simulink library "deadtime_with_minimum_pulse_generator"  (R2025b)
settings: Solver=VariableStepAuto  StartTime=0.0  StopTime=10.0  RelTol=1e-3
libraries: ee_lib x114, fl_lib x20, nesl_utility x5
(part 1 of 12)
settings Model: Creator=dbagn  LastModifiedBy=dbagn

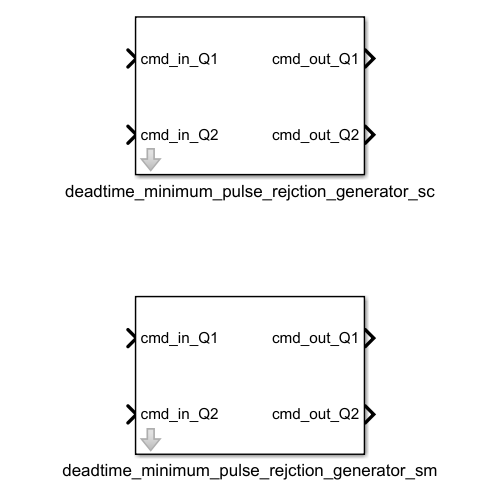
[thumbnail: Simulink's stored preview of the top-level diagram]
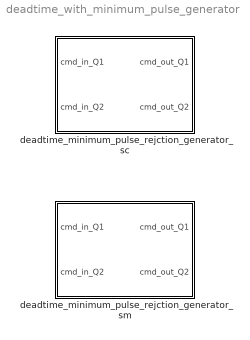
== system deadtime_with_minimum_pulse_generator ==
  deadtime_minimum_pulse_rejction_generator_sc : Subsystem  mask{Vpos_rail_dtg=15, Vneg_rail_dtg=0, Cdt=820e-12, Rdt=3.3e3, Cmp=270e-12, Rmp=3.3e3}
      mask prompts: Vpos_rail_dtg "Positive Voltage Rail Supply"; Vneg_rail_dtg "Negative Voltage Rail Supply"; Cdt "C dead time [F]"; Rdt "R dead time [Ohm]"; Cmp "C min pulse [F]"; Rmp "R min pulse [Ohm]"
  deadtime_minimum_pulse_rejction_generator_sm : Subsystem  mask{Vpos_rail_dtg=12, deadtime=2e-6, minimum_pulse=2e-6}
      mask prompts: Vpos_rail_dtg "Positive Voltage Rail Supply"; deadtime "DeadTime [s]"; minimum_pulse "Minimum Pulse [s]"

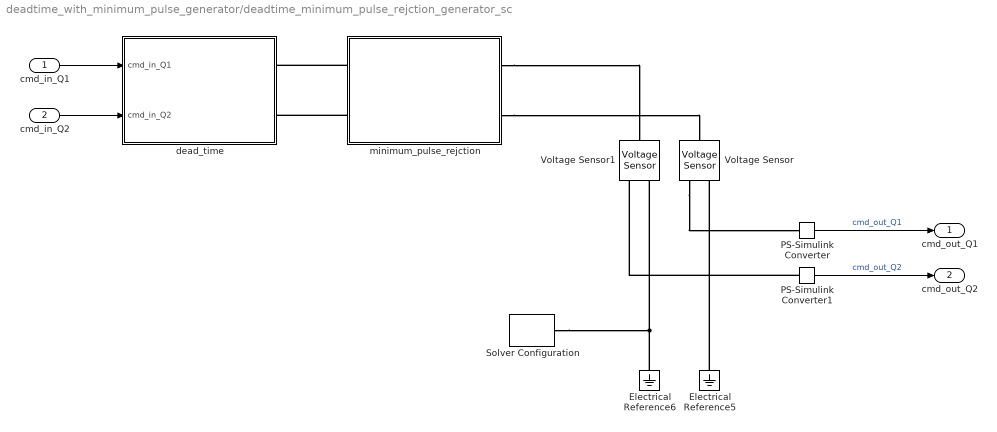
== system deadtime_with_minimum_pulse_generator/deadtime_minimum_pulse_rejction_generator_sc ==
  cmd_in_Q1 : Inport
  cmd_in_Q2 : Inport  Port=2
  Electrical Reference5 : fl_lib/Electrical/Electrical Elements/Electrical Reference
  Electrical Reference6 : fl_lib/Electrical/Electrical Elements/Electrical Reference
  PS-Simulink Converter : nesl_utility/PS-Simulink Converter  PhysicalDomain=network_engine_domain  SubClassName=ps_output  LeftPortType=input  RightPortType=output  PseudoPeriodic=off  Frequencies=[]  VectorFormat=1-D array  Unit=V  AffineConversion=off
  PS-Simulink Converter1 : nesl_utility/PS-Simulink Converter  PhysicalDomain=network_engine_domain  SubClassName=ps_output  LeftPortType=input  RightPortType=output  PseudoPeriodic=off  Frequencies=[]  VectorFormat=1-D array  Unit=V  AffineConversion=off
  Solver Configuration : nesl_utility/Solver Configuration  PhysicalDomain=network_engine_domain  SubClassName=solver  LeftPortType=input  RightPortType=generic  Tones=[]  Harmonics=[]  SimulateNoise=off  Profile=off  UseLocalSampling=off  EnableSwitchedLinearOptims=on  FrequencyDomain=off  UseCCode=off  RelTol=0.001  AbsTol=0.001  MinStep=1e-09  ToWorkspace=off  RevertToSquareIcSolve=off  NumHomotopyIterations=100  PhasorMode=off  PhasorModeNumHarmonics=1  ConsistencySolver=NEWTON_XTOL_AFTER_FTOL  IndexReductionMethod=DerivativeReplacement  DoDC=on  ResidualTolerance=1e-09  ConsistencyTolSource=GLOBAL  ConsistencyAbsTol=0.001  ConsistencyRelTol=0.001  ConsistencyTolFactor=0.001  UseLocalSolver=on  LocalSolverChoice=NE_BACKWARD_EULER_ADVANCER  ResolveIndetEquations=on  FunctionEvalNumThread=1  LocalSolverSampleTime=tc  DoFixedCost=off  MaxNonlinIter=5  MaxModeIter=2  ComputeImpulses=off  ImpulseIterations=2  LinearAlgebra=auto  LinearAlgebraNumThread=0  EquationFormulation=NE_TIME_EF  DelaysMemoryBudget=1024  AutomaticFiltering=on  FilteringTimeConstant=0.001  PartitionStorageMethod=AS_NEEDED  PartitionMemoryBudget=1024  PartitionMethod=ROBUST  MultibodyUseLocalSolver=off  MultibodyLocalSolverChoice=ODE1  MultibodyLocalSolverSampleTime=0.001
  Voltage Sensor : fl_lib/Electrical/Electrical Sensors/Voltage Sensor
  Voltage Sensor1 : fl_lib/Electrical/Electrical Sensors/Voltage Sensor
  dead_time : Subsystem
  minimum_pulse_rejction : Subsystem
  cmd_out_Q1 : Outport
  cmd_out_Q2 : Outport  Port=2
  wires:
  cmd_in_Q1/1 -> dead_time/1(cmd_in_Q1)
  cmd_in_Q2/1 -> dead_time/2(cmd_in_Q2)
  PS-Simulink Converter/1 -> cmd_out_Q1/1  "cmd_out_Q1"
  PS-Simulink Converter1/1 -> cmd_out_Q2/1  "cmd_out_Q2"
  connections:
  Electrical Reference6/LConn1 -- Voltage Sensor1/RConn2 -- Solver Configuration/RConn1
  Electrical Reference5/LConn1 -- Voltage Sensor/RConn2
  Voltage Sensor/RConn1 -- PS-Simulink Converter/LConn1
  PS-Simulink Converter1/LConn1 -- Voltage Sensor1/RConn1
  minimum_pulse_rejction/RConn1 -- Voltage Sensor1/LConn1
  minimum_pulse_rejction/RConn2 -- Voltage Sensor/LConn1
  minimum_pulse_rejction/LConn1 -- dead_time/RConn1
  minimum_pulse_rejction/LConn2 -- dead_time/RConn2

== system deadtime_with_minimum_pulse_generator/deadtime_minimum_pulse_rejction_generator_sm ==
  cmd_in_Q1 : Inport
  cmd_in_Q2 : Inport  Port=2
  dead_time : Subsystem
  minimum_pulse : Subsystem
  cmd_out_Q1 : Outport
  cmd_out_Q2 : Outport  Port=2
  wires:
  cmd_in_Q1/1 -> dead_time/1(cmd_in_Q1)
  cmd_in_Q2/1 -> dead_time/2(cmd_in_Q2)
  dead_time/1(cmd_out_Q1) -> minimum_pulse/1(cmd_in_Q1)
  dead_time/2(cmd_out_Q2) -> minimum_pulse/2(cmd_in_Q2)
  minimum_pulse/1(cmd_out_Q1) -> cmd_out_Q1/1
  minimum_pulse/2(cmd_out_Q2) -> cmd_out_Q2/1

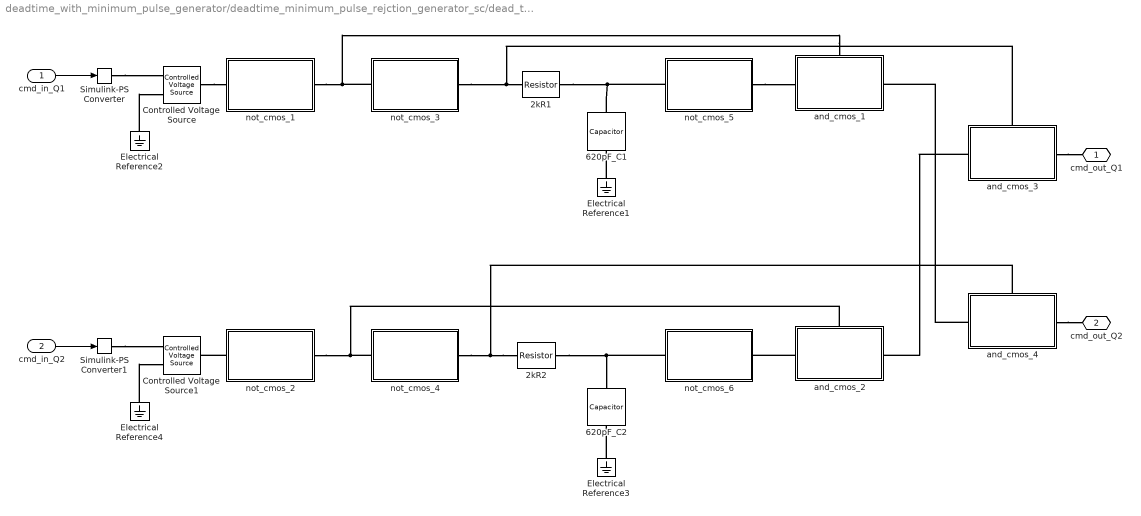
== system deadtime_with_minimum_pulse_generator/deadtime_minimum_pulse_rejction_generator_sc/dead_time ==
  cmd_in_Q1 : Inport
  cmd_in_Q2 : Inport  Port=2
  2kR1 : fl_lib/Electrical/Electrical Elements/Resistor  R=Rdt Ohm  i_specify=off  i_priority=None  i=0 A  i_nominal_specify=off  i_nominal_value=1  i_nominal_unit=A  v_specify=off  v_priority=None  v=0 V  v_nominal_specify=off  v_nominal_value=1  v_nominal_unit=V
  2kR2 : fl_lib/Electrical/Electrical Elements/Resistor  R=Rdt Ohm  i_specify=off  i_priority=None  i=0 A  i_nominal_specify=off  i_nominal_value=1  i_nominal_unit=A  v_specify=off  v_priority=None  v=0 V  v_nominal_specify=off  v_nominal_value=1  v_nominal_unit=V
  620pF_C1 : fl_lib/Electrical/Electrical Elements/Capacitor  c=Cdt F  r=1e-6 Ohm  g=0 1/Ohm  i_specify=off  i_priority=None  i=0 A  i_nominal_specify=off  i_nominal_value=1  i_nominal_unit=A  v_specify=off  v_priority=None  v=0 V  v_nominal_specify=off  v_nominal_value=1  v_nominal_unit=V  vc_specify=off  vc_priority=High  vc=0 V  vc_nominal_specify=off  vc_nominal_value=1  vc_nominal_unit=V
  620pF_C2 : fl_lib/Electrical/Electrical Elements/Capacitor  c=Cdt F  r=1e-6 Ohm  g=0 1/Ohm  i_specify=off  i_priority=None  i=0 A  i_nominal_specify=off  i_nominal_value=1  i_nominal_unit=A  v_specify=off  v_priority=None  v=0 V  v_nominal_specify=off  v_nominal_value=1  v_nominal_unit=V  vc_specify=off  vc_priority=High  vc=0 V  vc_nominal_specify=off  vc_nominal_value=1  vc_nominal_unit=V
  Controlled Voltage Source : fl_lib/Electrical/Electrical Sources/Controlled Voltage Source
  Controlled Voltage Source1 : fl_lib/Electrical/Electrical Sources/Controlled Voltage Source
  Electrical Reference{1..4} (4 alike) : fl_lib/Electrical/Electrical Elements/Electrical Reference
  Simulink-PS Converter : nesl_utility/Simulink-PS Converter  PhysicalDomain=network_engine_domain  SubClassName=ps_input  LeftPortType=input  RightPortType=output  PseudoPeriodic=off  Frequencies=[]  NoiseDistribution=none  NoiseParameters=[]  Unit=V  AffineConversion=off  FilteringAndDerivatives=provide  SimscapeFilterOrder=1  InputFilterTimeConstant=0.001  UdotUserProvided=0
  Simulink-PS Converter1 : nesl_utility/Simulink-PS Converter  PhysicalDomain=network_engine_domain  SubClassName=ps_input  LeftPortType=input  RightPortType=output  PseudoPeriodic=off  Frequencies=[]  NoiseDistribution=none  NoiseParameters=[]  Unit=V  AffineConversion=off  FilteringAndDerivatives=provide  SimscapeFilterOrder=1  InputFilterTimeConstant=0.001  UdotUserProvided=0
  and_cmos_1 : Subsystem
      settings: PortSchema="{\"entries\":[{\"content\":{\"sides\":[{\"content\":{\"connectorIds\":[\"LConn1\"]},\"type\":\"ConnectorPlacement.EquallySpacedRectSide\",\"uuid\":\"4468949f-f30a-49ce-949f-963bd607b697\"},{\"content\":{\"connectorIds\":[\"RConn1\"],\"side\":\"RIGHT\"},\"type\":\"ConnectorPlacement.EquallySpacedRectSide\",\"uuid\":\"ceda4040-901d-4fda-af9a-fc2c310617d8\"},{\"content\":{\"connectorIds\":[\"LConn2\"],\"side\":\"TOP\"},\"type\":\"ConnectorPlacement.EquallySpacedRectSide\",\"uuid\":\"3bda88a2-72eb-4af6-8d76-f1ae25008c8e\"}]},\"type\":\"ConnectorPlacement.EquallySpacedConnector\",\"uuid\":\"29371ddd-6b02-4938-80a9-3e3398458dce\"}],\"packageUris\":[\"http://schema.mathworks.com/mf0/Connector/R2020b\"],\"version\":\"1.0\"}"
  and_cmos_2 : Subsystem
      settings: PortSchema="{\"entries\":[{\"content\":{\"sides\":[{\"content\":{\"connectorIds\":[\"LConn1\"]},\"type\":\"ConnectorPlacement.EquallySpacedRectSide\",\"uuid\":\"4468949f-f30a-49ce-949f-963bd607b697\"},{\"content\":{\"connectorIds\":[\"RConn1\"],\"side\":\"RIGHT\"},\"type\":\"ConnectorPlacement.EquallySpacedRectSide\",\"uuid\":\"ceda4040-901d-4fda-af9a-fc2c310617d8\"},{\"content\":{\"connectorIds\":[\"LConn2\"],\"side\":\"TOP\"},\"type\":\"ConnectorPlacement.EquallySpacedRectSide\",\"uuid\":\"3bda88a2-72eb-4af6-8d76-f1ae25008c8e\"}]},\"type\":\"ConnectorPlacement.EquallySpacedConnector\",\"uuid\":\"29371ddd-6b02-4938-80a9-3e3398458dce\"}],\"packageUris\":[\"http://schema.mathworks.com/mf0/Connector/R2020b\"],\"version\":\"1.0\"}"
  and_cmos_3 : Subsystem
      settings: PortSchema="{\"entries\":[{\"content\":{\"sides\":[{\"content\":{\"connectorIds\":[\"LConn1\"]},\"type\":\"ConnectorPlacement.EquallySpacedRectSide\",\"uuid\":\"4468949f-f30a-49ce-949f-963bd607b697\"},{\"content\":{\"connectorIds\":[\"RConn1\"],\"side\":\"RIGHT\"},\"type\":\"ConnectorPlacement.EquallySpacedRectSide\",\"uuid\":\"ceda4040-901d-4fda-af9a-fc2c310617d8\"},{\"content\":{\"connectorIds\":[\"LConn2\"],\"side\":\"TOP\"},\"type\":\"ConnectorPlacement.EquallySpacedRectSide\",\"uuid\":\"3bda88a2-72eb-4af6-8d76-f1ae25008c8e\"}]},\"type\":\"ConnectorPlacement.EquallySpacedConnector\",\"uuid\":\"29371ddd-6b02-4938-80a9-3e3398458dce\"}],\"packageUris\":[\"http://schema.mathworks.com/mf0/Connector/R2020b\"],\"version\":\"1.0\"}"
  and_cmos_4 : Subsystem
      settings: PortSchema="{\"entries\":[{\"content\":{\"sides\":[{\"content\":{\"connectorIds\":[\"LConn1\"]},\"type\":\"ConnectorPlacement.EquallySpacedRectSide\",\"uuid\":\"4468949f-f30a-49ce-949f-963bd607b697\"},{\"content\":{\"connectorIds\":[\"RConn1\"],\"side\":\"RIGHT\"},\"type\":\"ConnectorPlacement.EquallySpacedRectSide\",\"uuid\":\"ceda4040-901d-4fda-af9a-fc2c310617d8\"},{\"content\":{\"connectorIds\":[\"LConn2\"],\"side\":\"TOP\"},\"type\":\"ConnectorPlacement.EquallySpacedRectSide\",\"uuid\":\"3bda88a2-72eb-4af6-8d76-f1ae25008c8e\"}]},\"type\":\"ConnectorPlacement.EquallySpacedConnector\",\"uuid\":\"29371ddd-6b02-4938-80a9-3e3398458dce\"}],\"packageUris\":[\"http://schema.mathworks.com/mf0/Connector/R2020b\"],\"version\":\"1.0\"}"
  not_cmos_1 : Subsystem
  not_cmos_2 : Subsystem
  not_cmos_3 : Subsystem
  not_cmos_4 : Subsystem
  not_cmos_5 : Subsystem
  not_cmos_6 : Subsystem
  cmd_out_Q1 : PMIOPort  Side=Right
  cmd_out_Q2 : PMIOPort  Port=2  Side=Right
  wires:
  cmd_in_Q2/1 -> Simulink-PS Converter1/1
  cmd_in_Q1/1 -> Simulink-PS Converter/1
  connections:
  2kR2/LConn1 -- and_cmos_4/LConn2 -- not_cmos_4/RConn1
  Electrical Reference1/LConn1 -- 620pF_C1/RConn1
  and_cmos_1/LConn2 -- not_cmos_3/LConn1 -- not_cmos_1/RConn1
  and_cmos_4/RConn1 -- cmd_out_Q2/RConn1
  2kR1/RConn1 -- not_cmos_5/LConn1 -- 620pF_C1/LConn1
  and_cmos_4/LConn1 -- and_cmos_1/RConn1
  and_cmos_2/LConn1 -- not_cmos_6/RConn1
  not_cmos_2/RConn1 -- and_cmos_2/LConn2 -- not_cmos_4/LConn1
  Electrical Reference4/LConn1 -- Controlled Voltage Source1/RConn2
  Electrical Reference3/LConn1 -- 620pF_C2/RConn1
  Simulink-PS Converter1/RConn1 -- Controlled Voltage Source1/RConn1
  2kR1/LConn1 -- and_cmos_3/LConn2 -- not_cmos_3/RConn1
  2kR2/RConn1 -- not_cmos_6/LConn1 -- 620pF_C2/LConn1
  not_cmos_5/RConn1 -- and_cmos_1/LConn1
  and_cmos_3/RConn1 -- cmd_out_Q1/RConn1
  not_cmos_2/LConn1 -- Controlled Voltage Source1/LConn1
  Electrical Reference2/LConn1 -- Controlled Voltage Source/RConn2
  Controlled Voltage Source/LConn1 -- not_cmos_1/LConn1
  and_cmos_3/LConn1 -- and_cmos_2/RConn1
  Simulink-PS Converter/RConn1 -- Controlled Voltage Source/RConn1

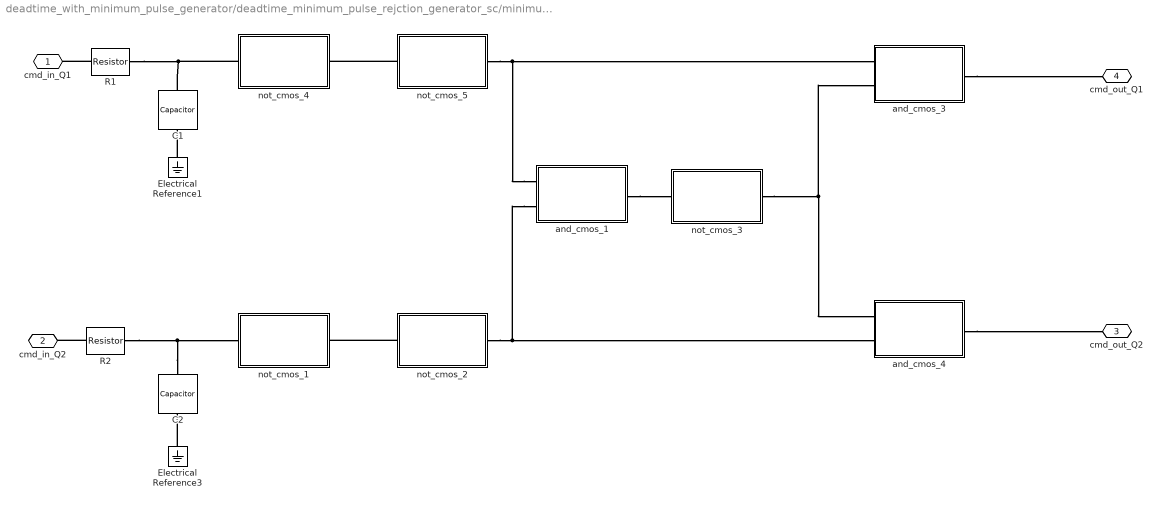
== system deadtime_with_minimum_pulse_generator/deadtime_minimum_pulse_rejction_generator_sc/minimum_pulse_rejction ==
  C1 : fl_lib/Electrical/Electrical Elements/Capacitor  c=Cmp F  r=1e-6 Ohm  g=0 1/Ohm  i_specify=off  i_priority=None  i=0 A  i_nominal_specify=off  i_nominal_value=1  i_nominal_unit=A  v_specify=off  v_priority=None  v=0 V  v_nominal_specify=off  v_nominal_value=1  v_nominal_unit=V  vc_specify=off  vc_priority=High  vc=0 V  vc_nominal_specify=off  vc_nominal_value=1  vc_nominal_unit=V
  C2 : fl_lib/Electrical/Electrical Elements/Capacitor  c=Cmp F  r=1e-6 Ohm  g=0 1/Ohm  i_specify=off  i_priority=None  i=0 A  i_nominal_specify=off  i_nominal_value=1  i_nominal_unit=A  v_specify=off  v_priority=None  v=0 V  v_nominal_specify=off  v_nominal_value=1  v_nominal_unit=V  vc_specify=off  vc_priority=High  vc=0 V  vc_nominal_specify=off  vc_nominal_value=1  vc_nominal_unit=V
  Electrical Reference1 : fl_lib/Electrical/Electrical Elements/Electrical Reference
  Electrical Reference3 : fl_lib/Electrical/Electrical Elements/Electrical Reference
  R1 : fl_lib/Electrical/Electrical Elements/Resistor  R=Rmp Ohm  i_specify=off  i_priority=None  i=0 A  i_nominal_specify=off  i_nominal_value=1  i_nominal_unit=A  v_specify=off  v_priority=None  v=0 V  v_nominal_specify=off  v_nominal_value=1  v_nominal_unit=V
  R2 : fl_lib/Electrical/Electrical Elements/Resistor  R=Rmp Ohm  i_specify=off  i_priority=None  i=0 A  i_nominal_specify=off  i_nominal_value=1  i_nominal_unit=A  v_specify=off  v_priority=None  v=0 V  v_nominal_specify=off  v_nominal_value=1  v_nominal_unit=V
  and_cmos_1 : Subsystem
  and_cmos_3 : Subsystem
  and_cmos_4 : Subsystem
  not_cmos_1 : Subsystem
  not_cmos_2 : Subsystem
  not_cmos_3 : Subsystem
  not_cmos_4 : Subsystem
  not_cmos_5 : Subsystem
  cmd_in_Q1 : PMIOPort  Side=Left
  cmd_in_Q2 : PMIOPort  Port=2  Side=Left
  cmd_out_Q2 : PMIOPort  Port=3  Side=Right
  cmd_out_Q1 : PMIOPort  Port=4  Side=Right
  connections:
  and_cmos_1/LConn1 -- and_cmos_3/LConn1 -- not_cmos_5/RConn1
  not_cmos_5/LConn1 -- not_cmos_4/RConn1
  and_cmos_1/RConn1 -- not_cmos_3/LConn1
  and_cmos_1/LConn2 -- and_cmos_4/LConn2 -- not_cmos_2/RConn1
  C2/LConn1 -- not_cmos_1/LConn1 -- R2/RConn1
  R1/RConn1 -- C1/LConn1 -- not_cmos_4/LConn1
  R1/LConn1 -- cmd_in_Q1/RConn1
  not_cmos_3/RConn1 -- and_cmos_4/LConn1 -- and_cmos_3/LConn2
  not_cmos_2/LConn1 -- not_cmos_1/RConn1
  Electrical Reference1/LConn1 -- C1/RConn1
  Electrical Reference3/LConn1 -- C2/RConn1
  and_cmos_3/RConn1 -- cmd_out_Q1/RConn1
  and_cmos_4/RConn1 -- cmd_out_Q2/RConn1
  R2/LConn1 -- cmd_in_Q2/RConn1

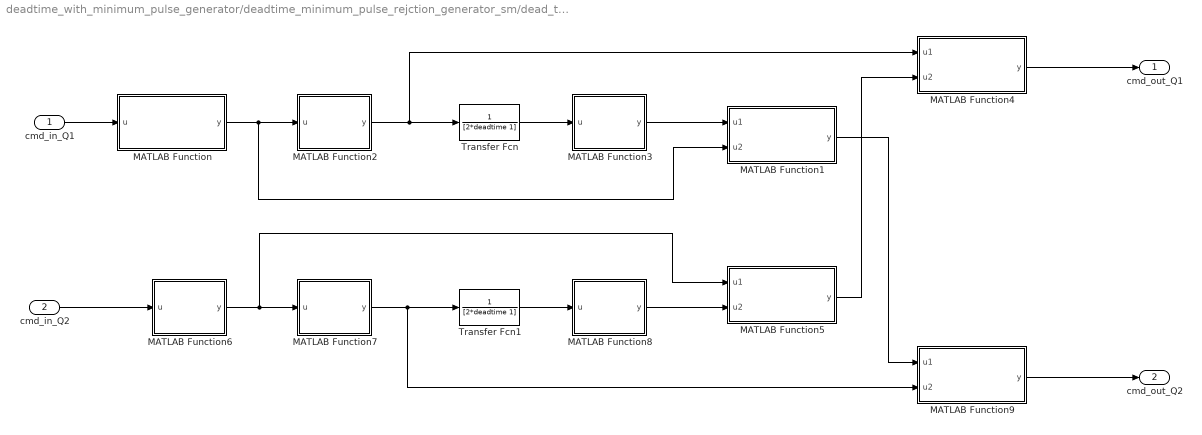
== system deadtime_with_minimum_pulse_generator/deadtime_minimum_pulse_rejction_generator_sm/dead_time ==
  cmd_in_Q1 : Inport
  cmd_in_Q2 : Inport  Port=2
  MATLAB Function : MATLAB Function  TreatAsAtomicUnit=on
  MATLAB Function1 : MATLAB Function  TreatAsAtomicUnit=on
  MATLAB Function2 : MATLAB Function  TreatAsAtomicUnit=on
  MATLAB Function3 : MATLAB Function  TreatAsAtomicUnit=on
  MATLAB Function4 : MATLAB Function  TreatAsAtomicUnit=on
  MATLAB Function5 : MATLAB Function  TreatAsAtomicUnit=on
  MATLAB Function6 : MATLAB Function  TreatAsAtomicUnit=on
  MATLAB Function7 : MATLAB Function  TreatAsAtomicUnit=on
  MATLAB Function8 : MATLAB Function  TreatAsAtomicUnit=on
  MATLAB Function9 : MATLAB Function  TreatAsAtomicUnit=on
  Transfer Fcn : TransferFcn  Denominator=[2*deadtime 1]
  Transfer Fcn1 : TransferFcn  Denominator=[2*deadtime 1]
  cmd_out_Q1 : Outport
  cmd_out_Q2 : Outport  Port=2
  wires:
  MATLAB Function/1(y) -> MATLAB Function1/2(u2), MATLAB Function2/1(u)
  MATLAB Function7/1(y) -> MATLAB Function9/2(u2), Transfer Fcn1/1
  MATLAB Function1/1(y) -> MATLAB Function9/1(u1)
  MATLAB Function8/1(y) -> MATLAB Function5/2(u2)
  cmd_in_Q1/1 -> MATLAB Function/1(u)
  cmd_in_Q2/1 -> MATLAB Function6/1(u)
  MATLAB Function3/1(y) -> MATLAB Function1/1(u1)
  MATLAB Function5/1(y) -> MATLAB Function4/2(u2)
  Transfer Fcn1/1 -> MATLAB Function8/1(u)
  MATLAB Function4/1(y) -> cmd_out_Q1/1
  Transfer Fcn/1 -> MATLAB Function3/1(u)
  MATLAB Function9/1(y) -> cmd_out_Q2/1
  MATLAB Function6/1(y) -> MATLAB Function7/1(u), MATLAB Function5/1(u1)
  MATLAB Function2/1(y) -> MATLAB Function4/1(u1), Transfer Fcn/1

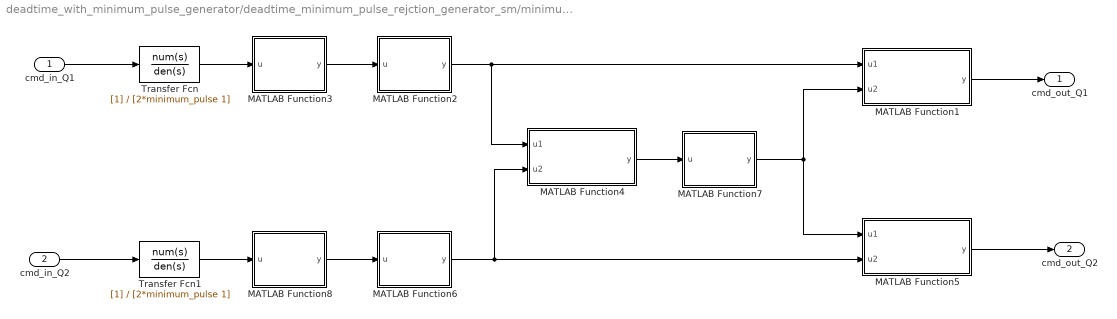
== system deadtime_with_minimum_pulse_generator/deadtime_minimum_pulse_rejction_generator_sm/minimum_pulse ==
  cmd_in_Q1 : Inport
  cmd_in_Q2 : Inport  Port=2
  MATLAB Function1 : MATLAB Function  TreatAsAtomicUnit=on
  MATLAB Function2 : MATLAB Function  TreatAsAtomicUnit=on
  MATLAB Function3 : MATLAB Function  TreatAsAtomicUnit=on
  MATLAB Function4 : MATLAB Function  TreatAsAtomicUnit=on
  MATLAB Function5 : MATLAB Function  TreatAsAtomicUnit=on
  MATLAB Function6 : MATLAB Function  TreatAsAtomicUnit=on
  MATLAB Function7 : MATLAB Function  TreatAsAtomicUnit=on
  MATLAB Function8 : MATLAB Function  TreatAsAtomicUnit=on
  Transfer Fcn : TransferFcn  Denominator=[2*minimum_pulse 1]
  Transfer Fcn1 : TransferFcn  Denominator=[2*minimum_pulse 1]
  cmd_out_Q1 : Outport
  cmd_out_Q2 : Outport  Port=2
  wires:
  Transfer Fcn/1 -> MATLAB Function3/1(u)
  Transfer Fcn1/1 -> MATLAB Function8/1(u)
  MATLAB Function3/1(y) -> MATLAB Function2/1(u)
  cmd_in_Q2/1 -> Transfer Fcn1/1
  cmd_in_Q1/1 -> Transfer Fcn/1
  MATLAB Function8/1(y) -> MATLAB Function6/1(u)
  MATLAB Function2/1(y) -> MATLAB Function1/1(u1), MATLAB Function4/1(u1)
  MATLAB Function6/1(y) -> MATLAB Function5/2(u2), MATLAB Function4/2(u2)
  MATLAB Function4/1(y) -> MATLAB Function7/1(u)
  MATLAB Function7/1(y) -> MATLAB Function1/2(u2), MATLAB Function5/1(u1)
  MATLAB Function1/1(y) -> cmd_out_Q1/1
  MATLAB Function5/1(y) -> cmd_out_Q2/1
